simulink model "gravityGradient"  (R2023b)
settings: Solver=VariableStepAuto  StartTime=0.0  StopTime=Tfinal  RelTol=1e-3
model workspace (MAT data in the model file):
  I_sim = [17509.8791644  0  0; 0  23616.372327  0; 0  0  36244.5798954]
libraries: matrix_library x2
settings Model: Creator=kristopherriordan  LastModifiedBy=annahylbert

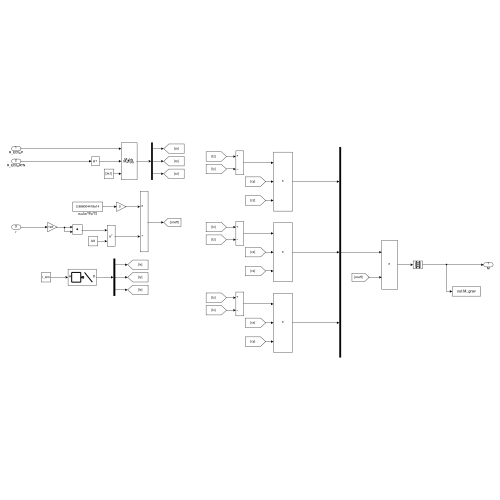
[thumbnail: Simulink's stored preview of the top-level diagram]
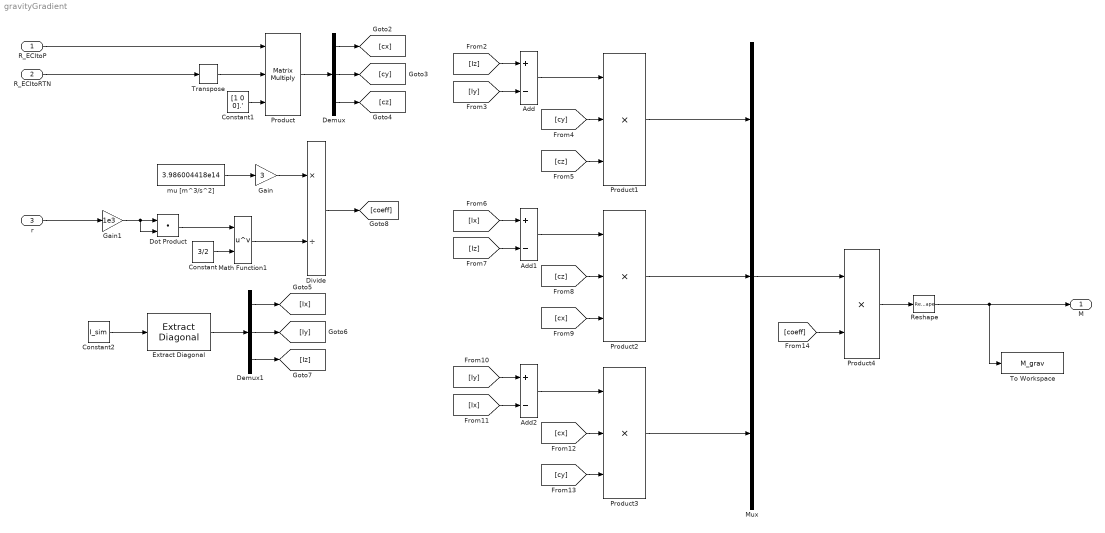
== system gravityGradient ==
  R_ECItoP : Inport  PortDimensions=[3 3]
  R_ECItoRTN : Inport  Port=2  PortDimensions=[3 3]
  r : Inport  Port=3  PortDimensions=[3 1]
  Add : Sum  Inputs=+-
  Add1 : Sum  Inputs=+-
  Add2 : Sum  Inputs=+-
  Constant : Constant  Value=3/2
  Constant1 : Constant  Value=[1 0 0].'  VectorParams1D=off
  Constant2 : Constant  Value=I_sim
  Demux : Demux  Outputs=3
  Demux1 : Demux  Outputs=3
  Divide : Product  Inputs=*/
  Dot Product : DotProduct  OutDataTypeStr=Inherit: Inherit via internal rule
  Extract Diagonal : matrix_library/Extract Diagonal
      settings: LibrarySourceBlock=|
      | simulink/Matrix
      | Operations/Extract Diagonal
  Gain : Gain  Gain=3
  Gain1 : Gain  Gain=1e3
  Math Function1 : Math  Operator=pow
  Mux : Mux  Inputs=3
  Product : Product  Inputs=***  Multiplication=Matrix(*)
  Product1 : Product  Inputs=***
  Product2 : Product  Inputs=***
  Product3 : Product  Inputs=***
  Product4 : Product
  Reshape : Reshape  OutputDimensionality=Column vector (2-D)
  To Workspace : ToWorkspace  VariableName=M_grav  SampleTime=-1
      settings: Save2DSignal=2-D array (concatenate along first dimension)
  Transpose : matrix_library/Transpose
  mu [m^3/s^2] : Constant  Value=3.986004418e14
  M : Outport
  wires:
  [Iy] -> Add/2
  [Iz] -> Add/1
  [cx] -> Product3/2
  Product2/1 -> Mux/2
  Demux1/2 -> [Iy]
  [coeff] -> Product4/2
  Product3/1 -> Mux/3
  Product4/1 -> Reshape/1
  [Ix] -> Add2/2
  Add2/1 -> Product3/1
  [cy] -> Product1/2
  R_ECItoRTN/1 -> Transpose/1
  Product1/1 -> Mux/1
  [cx] -> Product2/3
  Demux/3 -> [cz]
  Constant1/1 -> Product/3
  Demux/1 -> [cx]
  Demux1/1 -> [Ix]
  Mux/1 -> Product4/1
  R_ECItoP/1 -> Product/1
  Gain/1 -> Divide/1
  Add1/1 -> Product2/1
  Demux/2 -> [cy]
  Demux1/3 -> [Iz]
  Transpose/1 -> Product/2
  Extract Diagonal/1 -> Demux1/1
  [Iz] -> Add1/2
  Divide/1 -> [coeff]
  Add/1 -> Product1/1
  Math Function1/1 -> Divide/2
  [Ix] -> Add1/1
  Constant/1 -> Math Function1/2
  [cy] -> Product3/3
  [cz] -> Product1/3
  r/1 -> Gain1/1
  Dot Product/1 -> Math Function1/1
  Gain1/1 -> Dot Product/2, Dot Product/1
  [cz] -> Product2/2
  Reshape/1 -> To Workspace/1, M/1
  mu [m^3/s^2]/1 -> Gain/1
  Product/1 -> Demux/1
  [Iy] -> Add2/1
  Constant2/1 -> Extract Diagonal/1
